simulink model "autopilot"  (R2017a)
settings: Solver=VariableStepAuto  StartTime=0.0  StopTime=1000  RelTol=1e-3
values from neighbouring files (symbols this model uses):
  A = [-0.322     0.052   0.028   -1.12   0.002 ... (first row only)    [run_task_2f.m]
  B = [0; 0; 0; 0; 10]    [run_task_2f.m]
  C = [0 0 0 1 0 ... (first row only)    [run_task_2f.m]
  D = zeros(4, 1)    [run_task_2f.m]
  g = 9.81    [auoschmilot.m]    (also in run_task_2f.m)
  k_d_phi = (2*zeta_phi*w_n_phi-a_1)/a_2    [auoschmilot.m]    (also in run_task_2f.m)
  k_i_x = 0.195    [auoschmilot.m]    (also in run_task_2f.m)
  k_p_phi = -5/3    (= -1.66666666667)    [auoschmilot.m]    (also in run_task_2f.m)
  k_p_x = 2*zeta_X*w_n_x*V_g/g    [auoschmilot.m]    (also in run_task_2f.m)
  V_g = 637/3.6    (= 176.944444444)    [auoschmilot.m]    (also in run_task_2f.m)
libraries: simulink_extras x2
settings Model: Creator=rokru  LastModifiedBy=rokru

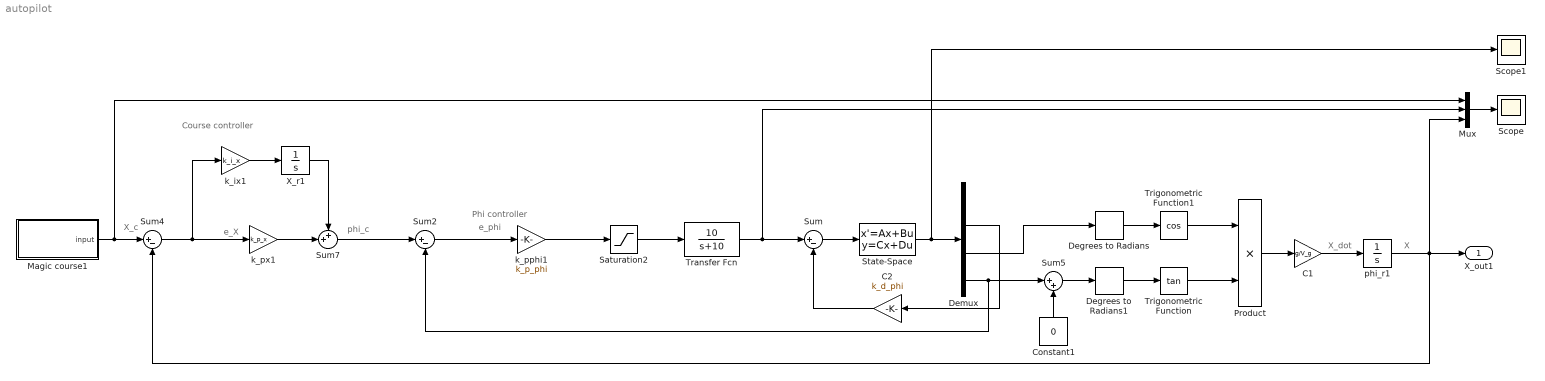
== system autopilot ==
  note: X
  note: X_c
  note: X_dot
  note: phi_c
  note: Course controller
  note: e_X
  note: Phi controller
  note: e_phi
  C1 : Gain  Gain=g/V_g
  C2 : Gain  Gain=k_d_phi
  Constant1 : Constant  Value=0
  Degrees to Radians : simulink_extras/Transformations/Degrees to Radians
  Degrees to Radians1 : simulink_extras/Transformations/Degrees to Radians
  Demux : Demux
  Magic course1 : Subsystem
  Mux : Mux  Inputs=3
  Product : Product
  Saturation2 : Saturate  UpperLimit=25  LowerLimit=-25
  Scope : Scope
  Scope1 : Scope
  State-Space : StateSpace  A=A  B=B  C=C  D=D  X0=0
  Sum : Sum  Inputs=|+-
  Sum2 : Sum  Inputs=|+-
  Sum4 : Sum  Inputs=|+-
  Sum5 : Sum  Inputs=|++
  Sum7 : Sum  Inputs=++|
  Transfer Fcn : TransferFcn  Numerator=[10]  Denominator=[1 10]
  Trigonometric Function : Trigonometry  Operator=tan
  Trigonometric Function1 : Trigonometry  Operator=cos
  X_r1 : Integrator
  k_ix1 : Gain  Gain=k_i_x
  k_pphi1 : Gain  Gain=k_p_phi
  k_px1 : Gain  Gain=k_p_x
  phi_r1 : Integrator
  X_out1 : Outport
  wires:
  State-Space/1 -> Scope1/1, Demux/1
  Trigonometric Function/1 -> Product/2
  C1/1 -> phi_r1/1
  k_px1/1 -> Sum7/2
  k_ix1/1 -> X_r1/1
  X_r1/1 -> Sum7/1
  Sum4/1 -> k_ix1/1, k_px1/1
  Magic course1/1(input) -> Mux/1, Sum4/1
  Product/1 -> C1/1
  C2/1 -> Sum/2
  Saturation2/1 -> Transfer Fcn/1
  phi_r1/1 -> Sum4/2, X_out1/1, Mux/3
  Mux/1 -> Scope/1
  Degrees to Radians1/1 -> Trigonometric Function/1
  Demux/3 -> Degrees to Radians/1
  Degrees to Radians/1 -> Trigonometric Function1/1
  Trigonometric Function1/1 -> Product/1
  Demux/2 -> C2/1
  Demux/4 -> Sum5/1, Sum2/2
  Sum/1 -> State-Space/1
  Constant1/1 -> Sum5/2
  Sum5/1 -> Degrees to Radians1/1
  k_pphi1/1 -> Saturation2/1
  Transfer Fcn/1 -> Sum/1, Mux/2
  Sum7/1 -> Sum2/1
  Sum2/1 -> k_pphi1/1

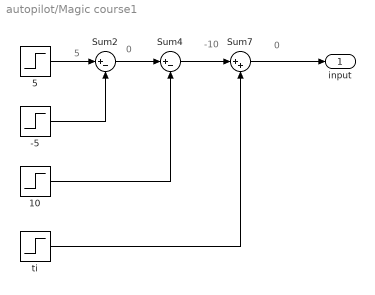
== system autopilot/Magic course1 ==
  note: 0
  note: -10
  note: 0
  note: 5
  -5 : Step  Time=100  After=5  SampleTime=0
  10 : Step  Time=150  After=10  SampleTime=0
  5 : Step  Time=10  After=5  SampleTime=0
  Sum2 : Sum  Inputs=|+-
  Sum4 : Sum  Inputs=|+-
  Sum7 : Sum  Inputs=|++
  ti : Step  Time=200  After=10  SampleTime=0
  input : Outport
  wires:
  10/1 -> Sum4/2
  ti/1 -> Sum7/2
  -5/1 -> Sum2/2
  Sum7/1 -> input/1
  5/1 -> Sum2/1
  Sum4/1 -> Sum7/1
  Sum2/1 -> Sum4/1
